simulink model "MBD_Assignment"  (R2022b)
settings: Solver=FixedStepAuto  StartTime=0.0  StopTime=10.0  RelTol=1e-3
undefined symbols (not defined in the file or in its folder): CurrentGear, StandPos
libraries: simulink x2
settings Model: Creator=prathmeshg  LastModifiedBy=prathmeshg
settings OptimizationCC: DefaultParameterBehavior=Inlined  EnhancedBackFolding=on  PassReuseOutputArgsAs=Individual arguments  ZeroExternalMemoryAtStartup=off  ZeroInternalMemoryAtStartup=off  OptimizeBlockOrder=speed  DifferentSizesBufferReuse=on  OptimizationCustomize=off  EfficientTunableParamExpr=on
settings DebuggingCC: ParameterTunabilityLossMsg=error
settings SFSimCC: MATLABDynamicMemAlloc=off
settings RTWCC: Description=AUTOSAR  SystemTargetFile=autosar.tlc  GenCodeOnly=on  TemplateMakefile=ert_default_tmf
settings CodeAppCC: ForceParamTrailComments=on  IgnoreCustomStorageClasses=off  OperatorAnnotations=on  SimulinkDataObjDesc=on  SFDataObjDesc=on  InsertBlockDesc=on
settings STFCustomTargetCC: TargetLangStandard=C99 (ISO)  MultiwordLength=256  ParMdlRefBuildCompliant=on  CompOptLevelCompliant=on  IncludeMdlTerminateFcn=off  CombineOutputUpdateFcns=on  SuppressErrorStatus=on  ERTCustomFileBanners=on  SupportNonFinite=off  SupportComplex=off  SupportContinuousTime=off  SupportNonInlinedSFcns=off  RemoveResetFunc=on  MATLABClassNameForMDSCustomization=Simulink.SoftwareTarget.ERTCustomization  AutosarCompliant=on  UseToolchainInfoCompliant=on  LookupTableObjectStructAxisOrder=2,1,3,4,...  LUTObjectStructOrderEvenSpacing=Size,Table,Breakpoints  SystemTargetFile=autosar.tlc
settings ERTTargetCC: TargetLangStandard=C99 (ISO)  ConcurrentExecutionCompliant=off  IncludeMdlTerminateFcn=off  SuppressErrorStatus=on  SupportNonFinite=off  SupportComplex=off  ModelStepFunctionPrototypeControlCompliant=off  CPPClassGenCompliant=off  AutosarCompliant=on  LookupTableObjectStructAxisOrder=2,1,3,4,...  LUTObjectStructOrderEvenSpacing=Size,Table,Breakpoints  InlinedParameterPlacement=NonHierarchical  ERTCustomFileTemplate=example_file_process.tlc

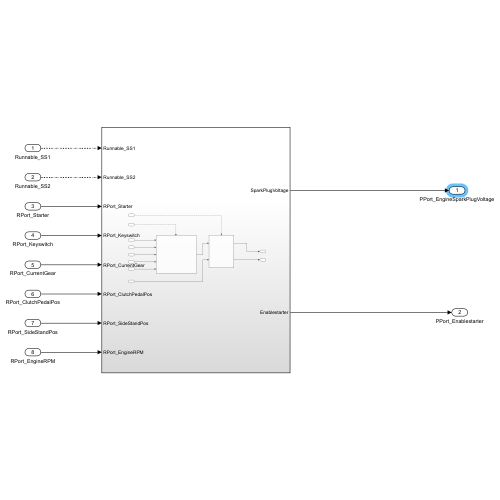
[thumbnail: Simulink's stored preview of the top-level diagram]
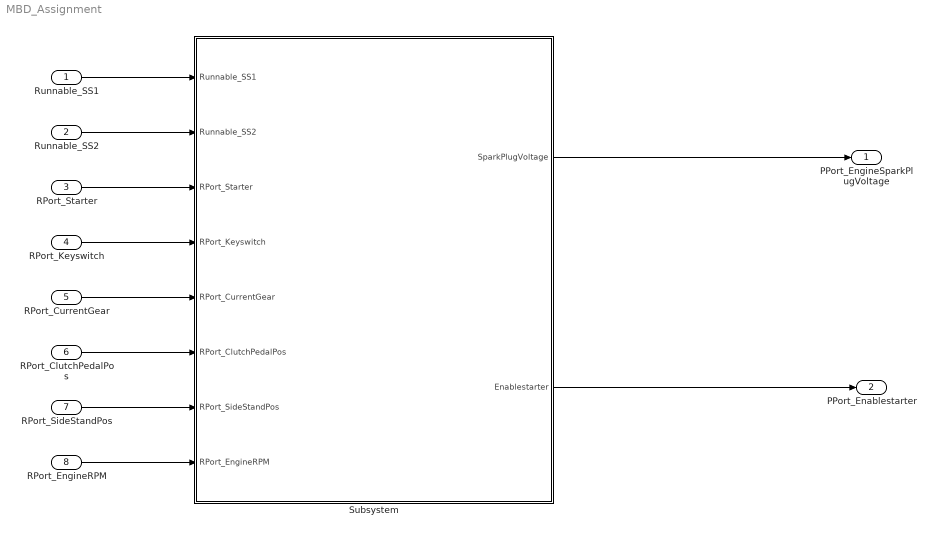
== system MBD_Assignment ==
  Runnable_SS1 : Inport  OutMin=[0]  OutMax=[100]  OutDataTypeStr=boolean  SampleTime=5  OutputFunctionCall=on
  Runnable_SS2 : Inport  Port=2  OutMin=[0]  OutMax=[100]  OutDataTypeStr=boolean  SampleTime=10  OutputFunctionCall=on
  RPort_Starter : Inport  Port=3  OutDataTypeStr=boolean
  RPort_Keyswitch : Inport  Port=4  OutDataTypeStr=boolean
  RPort_CurrentGear : Inport  Port=5  OutDataTypeStr=Enum: CurrentGear
  RPort_ClutchPedalPos : Inport  Port=6  OutMin=[0]  OutMax=[100]  OutDataTypeStr=int8
  RPort_SideStandPos : Inport  Port=7  OutDataTypeStr=Enum: StandPos
  RPort_EngineRPM : Inport  Port=8  OutDataTypeStr=uint32
  Subsystem : Subsystem
  PPort_EngineSparkPlugVoltage : Outport
  PPort_Enablestarter : Outport  Port=2
  wires:
  RPort_Keyswitch/1 -> Subsystem/4(RPort_Keyswitch)
  RPort_CurrentGear/1 -> Subsystem/5(RPort_CurrentGear)
  RPort_ClutchPedalPos/1 -> Subsystem/6(RPort_ClutchPedalPos)
  RPort_SideStandPos/1 -> Subsystem/7(RPort_SideStandPos)
  RPort_EngineRPM/1 -> Subsystem/8(RPort_EngineRPM)
  RPort_Starter/1 -> Subsystem/3(RPort_Starter)
  Subsystem/1(SparkPlugVoltage) -> PPort_EngineSparkPlugVoltage/1
  Runnable_SS2/1 -> Subsystem/2(Runnable_SS2)
  Runnable_SS1/1 -> Subsystem/1(Runnable_SS1)
  Subsystem/2(Enablestarter) -> PPort_Enablestarter/1

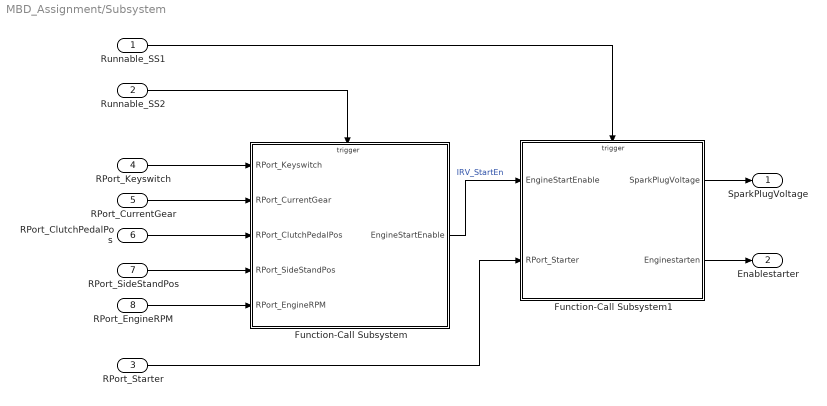
== system MBD_Assignment/Subsystem ==
  Runnable_SS1 : Inport  SampleTime=5
  Runnable_SS2 : Inport  Port=2  SampleTime=10
  RPort_Starter : Inport  Port=3
  RPort_Keyswitch : Inport  Port=4
  RPort_CurrentGear : Inport  Port=5
  RPort_ClutchPedalPos : Inport  Port=6
  RPort_SideStandPos : Inport  Port=7
  RPort_EngineRPM : Inport  Port=8
  Function-Call Subsystem : Subsystem  TreatAsAtomicUnit=on
  Function-Call Subsystem1 : Subsystem  TreatAsAtomicUnit=on
  SparkPlugVoltage : Outport
  Enablestarter : Outport  Port=2
  wires:
  RPort_CurrentGear/1 -> Function-Call Subsystem/2(RPort_CurrentGear)
  RPort_ClutchPedalPos/1 -> Function-Call Subsystem/3(RPort_ClutchPedalPos)
  RPort_SideStandPos/1 -> Function-Call Subsystem/4(RPort_SideStandPos)
  RPort_EngineRPM/1 -> Function-Call Subsystem/5(RPort_EngineRPM)
  Function-Call Subsystem/1(EngineStartEnable) -> Function-Call Subsystem1/1(EngineStartEnable)  "IRV_StartEn"
  Function-Call Subsystem1/1(SparkPlugVoltage) -> SparkPlugVoltage/1
  RPort_Keyswitch/1 -> Function-Call Subsystem/1(RPort_Keyswitch)
  Runnable_SS1/1 -> Function-Call Subsystem1/Trigger
  Runnable_SS2/1 -> Function-Call Subsystem/Trigger
  RPort_Starter/1 -> Function-Call Subsystem1/2(RPort_Starter)
  Function-Call Subsystem1/2(Enginestarten) -> Enablestarter/1

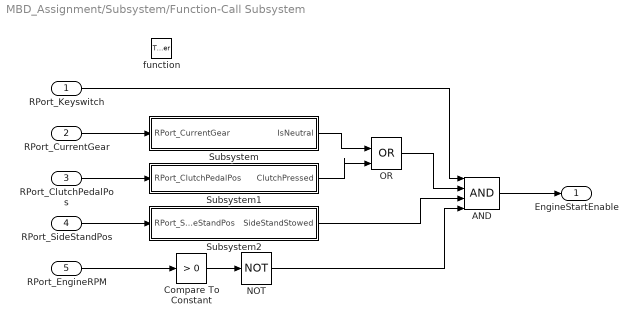
== system MBD_Assignment/Subsystem/Function-Call Subsystem ==
  RPort_Keyswitch : Inport
  RPort_CurrentGear : Inport  Port=2
  RPort_ClutchPedalPos : Inport  Port=3
  RPort_SideStandPos : Inport  Port=4
  RPort_EngineRPM : Inport  Port=5
  function : TriggerPort  TriggerType=function-call  VariantControl=(inherit)  SampleTimeType=periodic  SampleTime=-1
  AND : Logic  Inputs=4  IconShape=distinctive  AllPortsSameDT=off  OutDataTypeStr=boolean
  Compare To Constant : simulink/Logic and Bit Operations/Compare To Constant  relop=>  const=0  OutDataTypeStr=boolean
  NOT : Logic  Operator=NOT  IconShape=distinctive  AllPortsSameDT=off  OutDataTypeStr=boolean
  OR : Logic  Operator=OR  IconShape=distinctive  AllPortsSameDT=off  OutDataTypeStr=boolean
  Subsystem : Subsystem
  Subsystem1 : Subsystem
  Subsystem2 : Subsystem
  EngineStartEnable : Outport
  wires:
  RPort_CurrentGear/1 -> Subsystem/1(RPort_CurrentGear)
  RPort_ClutchPedalPos/1 -> Subsystem1/1(RPort_ClutchPedalPos)
  Subsystem/1(IsNeutral) -> OR/1
  Subsystem1/1(ClutchPressed) -> OR/2
  RPort_SideStandPos/1 -> Subsystem2/1(RPort_SideStandPos)
  RPort_EngineRPM/1 -> Compare To Constant/1
  Compare To Constant/1 -> NOT/1
  OR/1 -> AND/2
  Subsystem2/1(SideStandStowed) -> AND/3
  NOT/1 -> AND/4
  AND/1 -> EngineStartEnable/1
  RPort_Keyswitch/1 -> AND/1

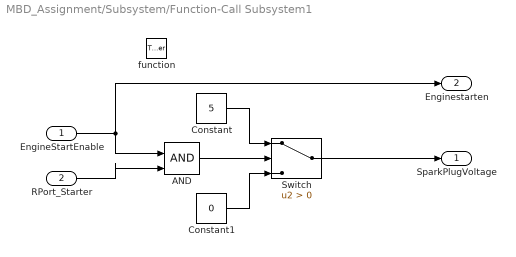
== system MBD_Assignment/Subsystem/Function-Call Subsystem1 ==
  EngineStartEnable : Inport
  RPort_Starter : Inport  Port=2
  function : TriggerPort  TriggerType=function-call  VariantControl=(inherit)  SampleTimeType=periodic  SampleTime=-1
  AND : Logic  IconShape=distinctive  AllPortsSameDT=off  OutDataTypeStr=boolean
  Constant : Constant  Value=5
  Constant1 : Constant  Value=0
  Switch : Switch  Criteria=u2 > Threshold  SaturateOnIntegerOverflow=off  InputSameDT=off
  SparkPlugVoltage : Outport
  Enginestarten : Outport  Port=2
  wires:
  EngineStartEnable/1 -> AND/1, Enginestarten/1
  RPort_Starter/1 -> AND/2
  AND/1 -> Switch/2
  Constant/1 -> Switch/1
  Constant1/1 -> Switch/3
  Switch/1 -> SparkPlugVoltage/1

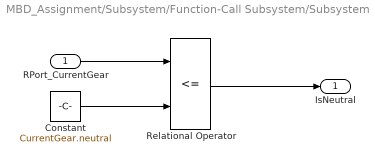
== system MBD_Assignment/Subsystem/Function-Call Subsystem/Subsystem ==
  RPort_CurrentGear : Inport
  Constant : Constant  Value=CurrentGear.neutral  OutDataTypeStr=Enum: CurrentGear
  Relational Operator : RelationalOperator  Operator=<=  OutDataTypeStr=boolean  RndMeth=Simplest  InputSameDT=off
  IsNeutral : Outport
  wires:
  RPort_CurrentGear/1 -> Relational Operator/1
  Constant/1 -> Relational Operator/2
  Relational Operator/1 -> IsNeutral/1

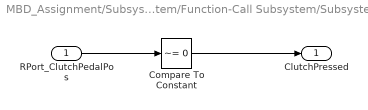
== system MBD_Assignment/Subsystem/Function-Call Subsystem/Subsystem1 ==
  RPort_ClutchPedalPos : Inport
  Compare To Constant : simulink/Logic and Bit Operations/Compare To Constant  relop=~=  const=0  OutDataTypeStr=boolean
  ClutchPressed : Outport
  wires:
  RPort_ClutchPedalPos/1 -> Compare To Constant/1
  Compare To Constant/1 -> ClutchPressed/1

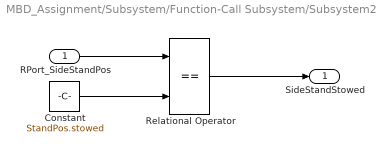
== system MBD_Assignment/Subsystem/Function-Call Subsystem/Subsystem2 ==
  RPort_SideStandPos : Inport
  Constant : Constant  Value=StandPos.stowed  OutDataTypeStr=Enum: StandPos
  Relational Operator : RelationalOperator  Operator===  OutDataTypeStr=boolean  RndMeth=Simplest  InputSameDT=off
  SideStandStowed : Outport
  wires:
  RPort_SideStandPos/1 -> Relational Operator/1
  Constant/1 -> Relational Operator/2
  Relational Operator/1 -> SideStandStowed/1
